simulink model "RCAMsimulink"  (R2024b)
settings: Solver=VariableStepAuto  StartTime=0.0  StopTime=TF  RelTol=1e-3
values from neighbouring files (symbols this model uses):
  x0 = [85 ... (first row only)    [sim_initialise.m]
undefined symbols (not defined in the file or in its folder): RCAM_model
settings Model: Creator=AAKRITI  LastModifiedBy=varsh

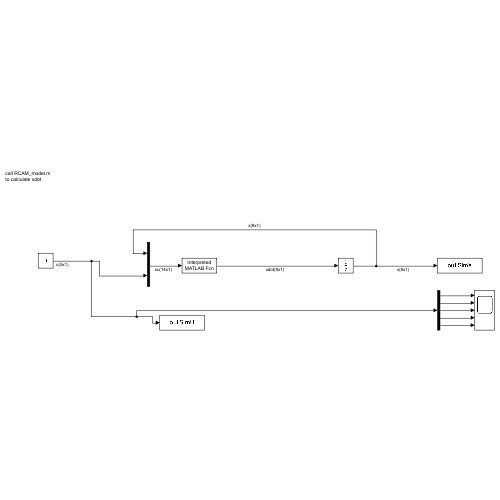
[thumbnail: Simulink's stored preview of the top-level diagram]
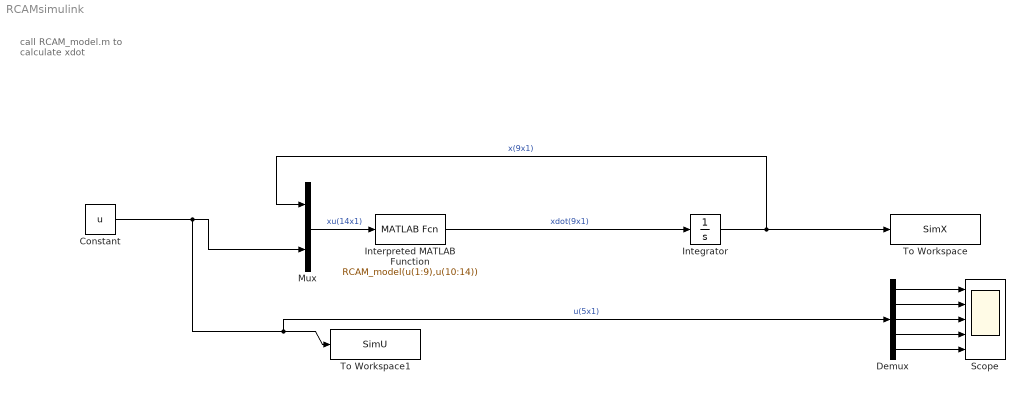
== system RCAMsimulink ==
  note: call RCAM_model.m
      | to calculate xdot
  Constant : Constant  Value=u
  Demux : Demux  Outputs=5
  Integrator : Integrator  InitialCondition=x0
  Interpreted MATLAB Function : MATLABFcn  MATLABFcn=RCAM_model(u(1:9),u(10:14))  OutputDimensions=9  Output1D=off
  Mux : Mux  Inputs=2
  Scope : Scope  NumInputPorts=5
  To Workspace : ToWorkspace  VariableName=SimX  SaveFormat=Timeseries  SampleTime=-1
  To Workspace1 : ToWorkspace  VariableName=SimU  SaveFormat=Timeseries  SampleTime=-1
  wires:
  Integrator/1 -> To Workspace/1, Mux/1  "x(9x1)"
  Interpreted MATLAB Function/1 -> Integrator/1  "xdot(9x1)"
  Constant/1 -> Demux/1, To Workspace1/1, Mux/2  "u(5x1)"
  Mux/1 -> Interpreted MATLAB Function/1  "xu(14x1)"
  Demux/1 -> Scope/1
  Demux/2 -> Scope/2
  Demux/3 -> Scope/3
  Demux/4 -> Scope/4
  Demux/5 -> Scope/5
